simulink model "ITireAppMdl"  (R2017b)
settings: Solver=FixedStepDiscrete  StartTime=0.0  StopTime=10000  FixedStep=0.1  RelTol=1e-3
model workspace (MAT data in the model file):
  AilrflowValidFlag1 = [0.01235 0.03834 0.06233 0.08839 0.11261 0.13833 0.16348 0.18843 0.2134 0.23767 0.26241 0.28847 ... (108920 elements, 54460x2)]
  AilrflowValidFlag2 = [0.01258 0.03858 0.06256 0.08863 0.11285 0.13856 0.16371 0.18866 0.21363 0.2379 0.26264 0.2887 ... (108920 elements, 54460x2)]
  Airflow = [0.01258 0.03858 0.06256 0.08863 0.11285 0.13856 0.16371 0.18866 0.21363 0.2379 0.26264 0.2887 ... (108920 elements, 54460x2)]
  Frequency = [0.01235 0.03834 0.06233 0.08839 0.11261 0.13833 0.16348 0.18843 0.2134 0.23767 0.26241 0.28847 ... (108920 elements, 54460x2)]
  IntkAirHmdty = [0.07576 0.17591 0.27589 0.37591 0.47621 0.5753 0.67605 0.77531 0.87537 0.97532 1.07528 1.17533 ... (27230 elements, 13615x2)]
  IntkAirTemp = [0.07576 0.17591 0.27589 0.37591 0.47621 0.5753 0.67605 0.77531 0.87537 0.97532 1.07528 1.17533 ... (27230 elements, 13615x2)]
  IntkHmdtyTemp = [0.07576 0.17591 0.27589 0.37591 0.47621 0.5753 0.67605 0.77531 0.87537 0.97532 1.07528 1.17533 ... (27230 elements, 13615x2)]
  PriPresFilterValue = [0.01235 0.03834 0.06233 0.08839 0.11261 0.13833 0.16348 0.18843 0.2134 0.23767 0.26241 0.28847 ... (108920 elements, 54460x2)]
  PriPresRawValue = [0.01235 0.03834 0.06233 0.08839 0.11261 0.13833 0.16348 0.18843 0.2134 0.23767 0.26241 0.28847 ... (108920 elements, 54460x2)]
  SecPresFilterValue = [0.01258 0.03858 0.06256 0.08863 0.11285 0.13856 0.16371 0.18866 0.21363 0.2379 0.26264 0.2887 ... (108920 elements, 54460x2)]
  SecPresRawValue = [0.01258 0.03858 0.06256 0.08863 0.11285 0.13856 0.16371 0.18866 0.21363 0.2379 0.26264 0.2887 ... (108920 elements, 54460x2)]
  deltaPriPresFilterV = [0.01235 0.03834 0.06233 0.08839 0.11261 0.13833 0.16348 0.18843 0.2134 0.23767 0.26241 0.28847 ... (108920 elements, 54460x2)]
  deltaPriPresRawValu = [0.01235 0.03834 0.06233 0.08839 0.11261 0.13833 0.16348 0.18843 0.2134 0.23767 0.26241 0.28847 ... (108920 elements, 54460x2)]
  deltaSecPresFilterV = [0.01258 0.03858 0.06256 0.08863 0.11285 0.13856 0.16371 0.18866 0.21363 0.2379 0.26264 0.2887 ... (108920 elements, 54460x2)]
  deltaSecPresRawValu = [0.01258 0.03858 0.06256 0.08863 0.11285 0.13856 0.16371 0.18866 0.21363 0.2379 0.26264 0.2887 ... (108920 elements, 54460x2)]
values from neighbouring files (symbols this model uses):
  pTireHighPreDWLimit = 335.0    [ITiremyDictionary.sldd]
  pTireHighPreUpLimit = 350.0    [ITiremyDictionary.sldd]
  pTireLowPreDWLimit = 180.0    [ITiremyDictionary.sldd]
  pTireLowPreUpLimit = 195.0    [ITiremyDictionary.sldd]
(part 2 of 2)

== stateflow chart ITireAppMdl/High_Low_PrsERR ==
  (default) -> (junction 814)
  (junction 814) -> (junction 815) [order 1] : [TireLFPrs>TireLFPrsRef]
  (junction 814) -> (junction 809) [order 2]
  (junction 815) -> (junction 813) : {TireLFPrsRef=TireLFPrs;
      | TireLFPrsSlowCounts=0;}
  (junction 813) -> (junction 809)
  (junction 809) -> (junction 802)
  (junction 802) -> (junction 807) [order 1] : [TireLRPrs>TireLRPrsRef]
  (junction 802) -> (junction 801) [order 2]
  (junction 807) -> (junction 800) : {TireLRPrsRef=TireLRPrs;
      | TireLRPrsSlowCounts=0;}
  (junction 800) -> (junction 801)
  (junction 801) -> (junction 792)
  (junction 792) -> (junction 798) [order 1] : [TireRFPrs>TireRFPrsRef]
  (junction 792) -> (junction 793) [order 2]
  (junction 798) -> (junction 795) : {TireRFPrsRef=TireRFPrs;
      | TireRFPrsSlowCounts=0;}
  (junction 795) -> (junction 793)
  (junction 793) -> (junction 783)
  (junction 783) -> (junction 785) [order 1] : [TireRRPrs>TireRRPrsRef]
  (junction 783) -> (junction 781) [order 2]
  (junction 785) -> (junction 787) : {TireRRPrsRef=TireRRPrs;
      | TireRRPrsSlowCounts=0;}
  (junction 787) -> (junction 781)
  (junction 781) -> (junction 148)
  (junction 148) -> (junction 152) [order 1] : [TireRFPrsV==0]
  (junction 152) -> (junction 174) [order 1] : [TireRFPrs>pTireLowPreUpLimit]
  (junction 148) -> (junction 150) [order 2] : {RFTirePreStaus=3;}
  (junction 152) -> (junction 158) [order 2]
  (junction 174) -> (junction 176) : {RFTirePreStaus=0;}
  (junction 176) -> (junction 158)
  (junction 158) -> (junction 210)
  (junction 210) -> (junction 213) [order 1] : [TireRFPrs<pTireHighPreDWLimit]
  (junction 210) -> (junction 208) [order 2]
  (junction 213) -> (junction 209) : {RFTirePreStaus=0;}
  (junction 209) -> (junction 208)
  (junction 208) -> (junction 222)
  (junction 222) -> (junction 225) [order 1] : [TireRFPrs<pTireLowPreDWLimit]
  (junction 222) -> (junction 220) [order 2]
  (junction 225) -> (junction 221) : {RFTirePreStaus=2;}
  (junction 221) -> (junction 220)
  (junction 220) -> (junction 226)
  (junction 226) -> (junction 233) [order 1] : [TireRFPrs>pTireHighPreUpLimit]
  (junction 226) -> (junction 231) [order 2]
  (junction 233) -> (junction 232) : {RFTirePreStaus=1;}
  (junction 231) -> (junction 150)
  (junction 232) -> (junction 231)
  (junction 150) -> (junction 242)
  (junction 242) -> (junction 241) [order 1] : [TireLFPrsV==0]
  (junction 241) -> (junction 256) [order 1] : [TireLFPrs>pTireLowPreUpLimit]
  (junction 242) -> (junction 240) [order 2] : {LFTirePreStaus=3;}
  (junction 241) -> (junction 276) [order 2]
  (junction 256) -> (junction 237) : {LFTirePreStaus=0;}
  (junction 237) -> (junction 276)
  (junction 276) -> (junction 251)
  (junction 251) -> (junction 254) [order 1] : [TireLFPrs<pTireHighPreDWLimit]
  (junction 251) -> (junction 249) [order 2]
  (junction 254) -> (junction 250) : {LFTirePreStaus=0;}
  (junction 250) -> (junction 249)
  (junction 249) -> (junction 258)
  (junction 258) -> (junction 265) [order 1] : [TireLFPrs<pTireLowPreDWLimit]
  (junction 258) -> (junction 263) [order 2]
  (junction 265) -> (junction 264) : {LFTirePreStaus=2;}
  (junction 264) -> (junction 263)
  (junction 263) -> (junction 267)
  (junction 267) -> (junction 274) [order 1] : [TireLFPrs>pTireHighPreUpLimit]
  (junction 267) -> (junction 272) [order 2]
  (junction 274) -> (junction 273) : {LFTirePreStaus=1;}
  (junction 272) -> (junction 240)
  (junction 273) -> (junction 272)
  (junction 240) -> (junction 285)
  (junction 285) -> (junction 284) [order 1] : [TireLRPrsV==0]
  (junction 284) -> (junction 289) [order 1] : [TireLRPrs>pTireLowPreUpLimit]
  (junction 285) -> (junction 280) [order 2] : {LRTirePreStaus=3;}
  (junction 284) -> (junction 306) [order 2]
  (junction 289) -> (junction 279) : {LRTirePreStaus=0}
  (junction 279) -> (junction 306)
  (junction 306) -> (junction 291)
  (junction 291) -> (junction 293) [order 1] : [TireLRPrs<pTireHighPreDWLimit]
  (junction 291) -> (junction 298) [order 2]
  (junction 293) -> (junction 295) : {LRTirePreStaus=0}
  (junction 295) -> (junction 298)
  (junction 298) -> (junction 300)
  (junction 300) -> (junction 315) [order 1] : [TireLRPrs<pTireLowPreDWLimit]
  (junction 300) -> (junction 313) [order 2]
  (junction 315) -> (junction 316) : {LRTirePreStaus=2}
  (junction 316) -> (junction 313)
  (junction 313) -> (junction 318)
  (junction 318) -> (junction 309) [order 1] : [TireLRPrs>pTireHighPreUpLimit]
  (junction 318) -> (junction 312) [order 2]
  (junction 309) -> (junction 307) : {LRTirePreStaus=1}
  (junction 312) -> (junction 280)
  (junction 307) -> (junction 312)
  (junction 280) -> (junction 327)
  (junction 327) -> (junction 326) [order 1] : [TireRRPrsV==0]
  (junction 326) -> (junction 334) [order 1] : [TireRRPrs>pTireLowPreUpLimit]
  (junction 327) -> (junction 322) [order 2] : {LRTirePreStaus=3;}
  (junction 326) -> (junction 348) [order 2]
  (junction 334) -> (junction 321) : {RRTirePreStaus=0}
  (junction 321) -> (junction 348)
  (junction 348) -> (junction 331)
  (junction 331) -> (junction 340) [order 1] : [TireRRPrs<pTireHighPreDWLimit]
  (junction 331) -> (junction 338) [order 2]
  (junction 340) -> (junction 337) : {RRTirePreStaus=0}
  (junction 337) -> (junction 338)
  (junction 338) -> (junction 342)
  (junction 342) -> (junction 352) [order 1] : [TireRRPrs<pTireLowPreDWLimit]
  (junction 342) -> (junction 356) [order 2]
  (junction 352) -> (junction 347) : {RRTirePreStaus=2}
  (junction 347) -> (junction 356)
  (junction 356) -> (junction 360)
  (junction 360) -> (junction 349) [order 1] : [TireRRPrs>pTireHighPreUpLimit]
  (junction 360) -> (junction 355) [order 2]
  (junction 349) -> (junction 358) : {RRTirePreStaus=1}
  (junction 355) -> (junction 322)
  (junction 358) -> (junction 355)
  (junction 322) -> (junction 362)
  (junction 362) -> (junction 543)
  (junction 543) -> (junction 545) : {Time1SCount++;}
  (junction 545) -> (junction 547) [order 1] : [Time1SCount>=60]
  (junction 545) -> (junction 687) [order 2]
  (junction 547) -> (junction 549) : {Time1SCount=0;
      | i=59;}
  (junction 549) -> (junction 557)
  (junction 561) -> (junction 549) [order 1] : [i>=1]
  (junction 557) -> (junction 559) : {LFPress1MinArray[i]=LFPress1MinArray[i-1];
      | LFPressV1MinArray[i]=LFPressV1MinArray[i-1];
      | i--;}
  (junction 559) -> (junction 561)
  (junction 561) -> (junction 566) [order 2] : {LFPress1MinArray[0]=TireLFPrs;
      | LFPressV1MinArray[0]=TireLFPrsV;
      | i=1;
      | }
  (junction 566) -> (junction 706) [order 1] : [(TireLFPrsV==0)]
  (junction 706) -> (junction 571)
  (junction 571) -> (junction 693) [order 1] : [((LFPress1MinArray[i]-LFPress1MinArray[0])>20)&(TireLFPrs>pTireLowPreDWLimit)]
  (junction 566) -> (junction 573) [order 2] : {LFTireLeakStaus=3;}
  (junction 715) -> (junction 706)
  (junction 571) -> (junction 708) [order 2] : {i++}
  (junction 693) -> (junction 701) : {LFTireLeakStaus=1;
      | TireLFPrsRef=TireLFPrs;
      | TireLFPrsSlowCounts=0;}
  (junction 708) -> (junction 715) [order 1] : [i<=59]
  (junction 708) -> (junction 703) [order 2] : {LFTireLeakStaus=0;}
  (junction 703) -> (junction 573)
  (junction 701) -> (junction 703)
  (junction 573) -> (junction 608) : {i=59;}
  (junction 608) -> (junction 611)
  (junction 609) -> (junction 608) [order 1] : [i>=1]
  (junction 611) -> (junction 613) : {LRPress1MinArray[i]=LRPress1MinArray[i-1];
      | LRPressV1MinArray[i]=LRPressV1MinArray[i-1];
      | i--;}
  (junction 613) -> (junction 609)
  (junction 609) -> (junction 605) [order 2] : {LRPress1MinArray[0]=TireLRPrs;
      | LRPressV1MinArray[0]=TireLRPrsV;
      | i=1;}
  (junction 605) -> (junction 724) [order 1] : [(TireLRPrsV==0)]
  (junction 724) -> (junction 722)
  (junction 722) -> (junction 735) [order 1] : [((LRPress1MinArray[i]-LRPress1MinArray[0])>20)&(TireLRPrs>pTireLowPreDWLimit)]
  (junction 605) -> (junction 600) [order 2] : {LRTireLeakStaus=3;}
  (junction 732) -> (junction 724)
  (junction 722) -> (junction 727) [order 2] : {i++}
  (junction 735) -> (junction 734) : {LRTireLeakStaus=1;
      | TireLRPrsRef=TireLRPrs;
      | TireLRPrsSlowCounts=0;}
  (junction 727) -> (junction 732) [order 1] : [i<=59]
  (junction 727) -> (junction 725) [order 2] : {LRTireLeakStaus=0;}
  (junction 734) -> (junction 725)
  (junction 725) -> (junction 600)
  (junction 600) -> (junction 634) : {i=59;}
  (junction 634) -> (junction 637)
  (junction 635) -> (junction 634) [order 1] : [i>=1]
  (junction 637) -> (junction 639) : {RFPress1MinArray[i]=RFPress1MinArray[i-1];
      | RFPressV1MinArray[i]=RFPressV1MinArray[i-1];
      | i--;}
  (junction 639) -> (junction 635)
  (junction 635) -> (junction 631) [order 2] : {RFPress1MinArray[0]=TireRFPrs;
      | RFPressV1MinArray[0]=TireRFPrsV;
      | i=1;}
  (junction 631) -> (junction 744) [order 1] : [(TireRFPrsV==0)]
  (junction 744) -> (junction 739)
  (junction 739) -> (junction 749) [order 1] : [((RFPress1MinArray[i]-RFPress1MinArray[0])>20)&(TireRFPrs>pTireLowPreDWLimit)]
  (junction 631) -> (junction 626) [order 2] : {RFTireLeakStaus=3;}
  (junction 752) -> (junction 744)
  (junction 739) -> (junction 746) [order 2] : {i++}
  (junction 749) -> (junction 751) : {RFTireLeakStaus=1;
      | TireRFPrsRef=TireRFPrs;
      | TireRFPrsSlowCounts=0;}
  (junction 746) -> (junction 752) [order 1] : [i<=59]
  (junction 746) -> (junction 742) [order 2] : {RFTireLeakStaus=0;}
  (junction 751) -> (junction 742)
  (junction 742) -> (junction 626)
  (junction 626) -> (junction 647) : {i=59;}
  (junction 647) -> (junction 663)
  (junction 661) -> (junction 647) [order 1] : [i>=1]
  (junction 663) -> (junction 665) : {RRPress1MinArray[i]=RRPress1MinArray[i-1];
      | RRPressV1MinArray[i]=RRPressV1MinArray[i-1];
      | i--;}
  (junction 665) -> (junction 661)
  (junction 661) -> (junction 657) [order 2] : {RRPress1MinArray[0]=TireRRPrs;
      | RRPressV1MinArray[0]=TireRRPrsV;}
  (junction 657) -> (junction 767) [order 1] : [(TireRRPrsV==0)]
  (junction 767) -> (junction 757)
  (junction 757) -> (junction 768) [order 1] : [((RRPress1MinArray[i]-RRPress1MinArray[0])>20)&(TireRRPrs>pTireLowPreDWLimit)]
  (junction 657) -> (junction 652) [order 2] : {RRTireLeakStaus=3;}
  (junction 760) -> (junction 767)
  (junction 757) -> (junction 765) [order 2] : {i++}
  (junction 768) -> (junction 759) : {RRTireLeakStaus=1;
      | TireRRPrsRef=TireRRPrs;
      | TireRRPrsSlowCounts=0;}
  (junction 765) -> (junction 760) [order 1] : [i<=59]
  (junction 765) -> (junction 769) [order 2] : {RRTireLeakStaus=0;}
  (junction 759) -> (junction 769)
  (junction 769) -> (junction 652)
  (junction 652) -> (junction 673)
  (junction 673) -> (junction 818) [order 1] : [(TireLFPrs<=TireLFPrsRef)&&(LFTireLeakStaus==0)]
  (junction 673) -> (junction 836) [order 2]
  (junction 818) -> (junction 820) : {TireLFPrsSlowCounts++;}
  (junction 820) -> (junction 824) [order 1] : [(TireLFPrsSlowCounts<36000)&&((TireLFPrsRef-TireLFPrs)>25)&&(TireLFPrs>pTireLowPreDWLimit)]
  (junction 820) -> (junction 826) [order 2] : {LFTireLeakStaus=0;}
  (junction 824) -> (junction 828) : {LFTireLeakStaus=2;
      | TireSlowLifeLF=((TireLFPrsRef-pTireLowPreDWLimit)/(TireLFPrsRef-TireLFPrs))*(TireLFPrsSlowCounts/600);}
  (junction 826) -> (junction 831) [order 1] : [(TireLFPrsSlowCounts>=36000)]
  (junction 826) -> (junction 839) [order 2]
  (junction 831) -> (junction 832) : {TireLFPrsSlowCounts=0;
      | TireLFPrsRef=TireLFPrs}
  (junction 839) -> (junction 836)
  (junction 832) -> (junction 839)
  (junction 828) -> (junction 832)
  (junction 836) -> (junction 843)
  (junction 843) -> (junction 853) [order 1] : [(TireLRPrs<=TireLRPrsRef)&(LRTireLeakStaus==0)]
  (junction 843) -> (junction 852) [order 2]
  (junction 853) -> (junction 848) : {TireLRPrsSlowCounts++;}
  (junction 848) -> (junction 865) [order 1] : [(TireLRPrsSlowCounts<36000)&((TireLRPrsRef-TireLRPrs)>25)&(TireLRPrs>pTireLowPreDWLimit)]
  (junction 848) -> (junction 850) [order 2] : {LRTireLeakStaus=0}
  (junction 865) -> (junction 847) : {LRTireLeakStaus=2;
      | TireSlowLifeLR=((TireLRPrsRef-pTireLowPreDWLimit)/(TireLRPrsRef-TireLRPrs))*(TireLRPrsSlowCounts/600);}
  (junction 850) -> (junction 857) [order 1] : [(TireLRPrsSlowCounts>=36000)]
  (junction 850) -> (junction 846) [order 2]
  (junction 857) -> (junction 862) : {TireLRPrsSlowCounts=0;
      | TireLRPrsRef=TireLFPrs}
  (junction 846) -> (junction 852)
  (junction 862) -> (junction 846)
  (junction 847) -> (junction 862)
  (junction 852) -> (junction 868)
  (junction 868) -> (junction 875) [order 1] : [(TireRFPrs<=TireRFPrsRef)&(RFTireLeakStaus==0)]
  (junction 868) -> (junction 882) [order 2]
  (junction 875) -> (junction 866) : {TireRFPrsSlowCounts++}
  (junction 866) -> (junction 887) [order 1] : [(TireRFPrsSlowCounts<36000)&((TireRFPrsRef-TireRFPrs)>25)&(TireRFPrs>pTireLowPreDWLimit)]
  (junction 866) -> (junction 873) [order 2] : {RFTireLeakStaus=0}
  (junction 887) -> (junction 870) : {RFTireLeakStaus=2;
      | TireSlowLifeRF=((TireRFPrsRef-pTireLowPreDWLimit)/(TireRFPrsRef-TireRFPrs))*(TireRFPrsSlowCounts/600);}
  (junction 873) -> (junction 878) [order 1] : [(TireRFPrsSlowCounts>=36000)]
  (junction 873) -> (junction 869) [order 2]
  (junction 878) -> (junction 872) : {TireRFPrsSlowCounts=0;
      | TireRFPrsRef=TireLFPrs}
  (junction 869) -> (junction 882)
  (junction 872) -> (junction 869)
  (junction 870) -> (junction 872)
  (junction 882) -> (junction 894)
  (junction 894) -> (junction 893) [order 1] : [(TireRRPrs<=TireRRPrsRef)&(RRTireLeakStaus==0)]
  (junction 894) -> (junction 904) [order 2]
  (junction 893) -> (junction 889) : {TireRRPrsSlowCounts++}
  (junction 889) -> (junction 910) [order 1] : [(TireRRPrsSlowCounts<36000)&((TireRRPrsRef-TireRRPrs)>25)&(TireRRPrs>pTireLowPreDWLimit)]
  (junction 889) -> (junction 895) [order 2] : {RRTireLeakStaus=0 }
  (junction 910) -> (junction 897) : {RRTireLeakStaus=2;
      | TireSlowLifeRR=((TireRRPrsRef-pTireLowPreDWLimit)/(TireRRPrsRef-TireRRPrs))*(TireRRPrsSlowCounts/600);}
  (junction 895) -> (junction 901) [order 1] : [(TireRRPrsSlowCounts>=36000)]
  (junction 895) -> (junction 898) [order 2]
  (junction 901) -> (junction 896) : {TireRRPrsSlowCounts=0;
      | TireRRPrsRef=TireLFPrs;}
  (junction 904) -> (junction 687)
  (junction 898) -> (junction 904)
  (junction 896) -> (junction 898)
  (junction 897) -> (junction 896)
  data: TireRFPrsV input uint8 [0..1]; TireLFPrsV input uint8 [0..1]; TireRRPrsV input uint8 [0..1]; TireLRPrsV input uint8 [0..1]; TireLFPrs input uint16 [0..1]; TireLRPrs input uint16 [0..1]; TireRFPrs input uint16 [0..1]; TireRRPrs input uint16 [0..1]; pTireHighPreUpLimit parameter double; pTireHighPreDWLimit parameter double; pTireLowPreUpLimit parameter double; pTireLowPreDWLimit parameter double; RFTirePreStaus output uint8; LFTirePreStaus output uint8; LRTirePreStaus output uint8; RRTirePreStaus output uint8; LFTireLeakStaus output uint8 =0; LRTireLeakStaus output uint8 =0; RFTireLeakStaus output uint8 =0; RRTireLeakStaus output uint8 =0; LFPress1MinArray local uint16 size=[1 60] =0; Time1SCount local uint8 =10; i local uint8 =0; LFPressV1MinArray local uint8 size=[1 60] =0; LRPressV1MinArray local uint8 size=[1 60] =0; RFPressV1MinArray local uint8 size=[1 60] =0; RRPressV1MinArray local uint8 size=[1 60] =0; RFPress1MinArray local uint16 size=[1 60] =0; LRPress1MinArray local uint16 size=[1 60] =0; RRPress1MinArray local uint16 size=[1 60] =0; TireLFPrsRef local uint16 [0..1] =0; TireLRPrsRef local uint16 [0..1] =0; TireRFPrsRef local uint16 [0..1] =0; TireRRPrsRef local uint16 [0..1] =0; TireLFPrsSlowCounts local uint16 [0..1] =0; TireLRPrsSlowCounts local uint16 [0..1] =0; TireRRPrsSlowCounts local uint16 [0..1] =0; TireSlowLifeLF output uint8; TireRFPrsSlowCounts local uint16 [0..1] =0; TireSlowLifeLR output uint8; TireSlowLifeRF output uint8; TireSlowLifeRR output uint8

== stateflow chart ITireAppMdl/TireTempStatus ==
  (default) -> (junction 13)
  (junction 13) -> (junction 19) [order 1] : [TireLFTmpV==0]
  (junction 19) -> (junction 21) [order 1] : [TireLFTmp>70]
  (junction 13) -> (junction 17) [order 2] : {LFTireTempStaus=3;}
  (junction 19) -> (junction 24) [order 2] : {LFTireTempStaus=0;}
  (junction 21) -> (junction 25) : {LFTireTempStaus=1;}
  (junction 24) -> (junction 17)
  (junction 25) -> (junction 24)
  (junction 17) -> (junction 30)
  (junction 30) -> (junction 33) [order 1] : [TireLRTmpV==0]
  (junction 33) -> (junction 42) [order 1] : [TireLRTmp>70]
  (junction 30) -> (junction 36) [order 2] : {LRTireTempStaus=3;}
  (junction 33) -> (junction 37) [order 2] : {LRTireTempStaus=0;}
  (junction 42) -> (junction 43) : {LRTireTempStaus=1;}
  (junction 37) -> (junction 36)
  (junction 43) -> (junction 37)
  (junction 36) -> (junction 48)
  (junction 48) -> (junction 55) [order 1] : [TireRFTmpV==0]
  (junction 55) -> (junction 51) [order 1] : [TireRFTmp>70]
  (junction 48) -> (junction 58) [order 2] : {RFTireTempStaus=3;}
  (junction 55) -> (junction 45) [order 2] : {RFTireTempStaus=0;}
  (junction 51) -> (junction 46) : {RFTireTempStaus=1;}
  (junction 45) -> (junction 58)
  (junction 46) -> (junction 45)
  (junction 58) -> (junction 66)
  (junction 66) -> (junction 70) [order 1] : [TireRRTmpV==0]
  (junction 70) -> (junction 67) [order 1] : [TireRRTmp>70]
  (junction 66) -> (junction 72) [order 2] : {RRTireTempStaus=3;}
  (junction 70) -> (junction 61) [order 2] : {RRTireTempStaus=0;}
  (junction 67) -> (junction 60) : {RRTireTempStaus=1;}
  (junction 61) -> (junction 72)
  (junction 60) -> (junction 61)
  (junction 72) -> (junction 75)
  data: TireLFTmpV input uint8; TireLFTmp input int16; TireLRTmpV input uint8; TireLRTmp input int16; TireRFTmpV input uint8; TireRFTmp input int16; TireRRTmpV input uint8; TireRRTmp input int16; LFTireTempStaus output uint8; LRTireTempStaus output uint8; RFTireTempStaus output uint8; RRTireTempStaus output uint8; data local double

== stateflow chart ITireAppMdl/SensorLostERR ==
  (default) -> (junction 16)
  (junction 16) -> (junction 22) [order 2] : {LFTirPreSenLostErrV=0;
      | LRTirPreSenLostErrV=0;RFTirPreSenLostErrV=0;
      | RRTirPreSenLostErrV=0;}
  (junction 22) -> (junction 26) [order 2] : {TireRFPrsLostCount=0;}
  (junction 16) -> (junction 18) [order 1] : [(VehSpdAvgNDrvn<37)||(VehSpdAvgNDrvnV==1)]{LFTirPreSenLostErrV=1;
      | LRTirPreSenLostErrV=1;RFTirPreSenLostErrV=1;
      | RRTirPreSenLostErrV=1;}
  (junction 22) -> (junction 24) [order 1] : [TireRFPrsV==1]{TireRFPrsLostCount = TireRFPrsLostCount + 1;}
  (junction 26) -> (junction 28)
  (junction 28) -> (junction 24)
  (junction 24) -> (junction 33)
  (junction 33) -> (junction 118) [order 2] : {TireLFPrsLostCount=0;}
  (junction 33) -> (junction 47) [order 1] : [TireLFPrsV==1]{TireLFPrsLostCount = TireLFPrsLostCount + 1;}
  (junction 118) -> (junction 120)
  (junction 120) -> (junction 47)
  (junction 47) -> (junction 55)
  (junction 55) -> (junction 129) [order 2] : {TireLRPrsLostCount=0;}
  (junction 55) -> (junction 63) [order 1] : [TireLRPrsV==1]{TireLRPrsLostCount = TireLRPrsLostCount + 1;}
  (junction 129) -> (junction 130)
  (junction 130) -> (junction 63)
  (junction 63) -> (junction 70)
  (junction 70) -> (junction 134) [order 2] : {TireRRPrsLostCount=0;}
  (junction 70) -> (junction 69) [order 1] : [TireRRPrsV==1]{TireRRPrsLostCount = TireRRPrsLostCount + 1;}
  (junction 134) -> (junction 135)
  (junction 135) -> (junction 69)
  (junction 69) -> (junction 73)
  (junction 73) -> (junction 77) [order 2] : {RFTirPreSenLostErr=0;}
  (junction 73) -> (junction 75) [order 1] : [TireRFPrsLostCount>pTirePrsLostCountTh]{RFTirPreSenLostErr=1;
      | TireRFPrsLostCount=pTirePrsLostCountTh}
  (junction 77) -> (junction 79)
  (junction 79) -> (junction 75)
  (junction 75) -> (junction 84)
  (junction 84) -> (junction 82) [order 2] : {LFTirPreSenLostErr=0;}
  (junction 84) -> (junction 90) [order 1] : [TireLFPrsLostCount>pTirePrsLostCountTh]{LFTirPreSenLostErr=1;
      | TireLFPrsLostCount=pTirePrsLostCountTh}
  (junction 82) -> (junction 88)
  (junction 88) -> (junction 90)
  (junction 90) -> (junction 98)
  (junction 98) -> (junction 99) [order 2] : {LRTirPreSenLostErr=0;}
  (junction 98) -> (junction 92) [order 1] : [TireLRPrsLostCount>pTirePrsLostCountTh]{LRTirPreSenLostErr=1;
      | TireLRPrsLostCount=pTirePrsLostCountTh}
  (junction 99) -> (junction 93)
  (junction 93) -> (junction 92)
  (junction 92) -> (junction 107)
  (junction 107) -> (junction 102) [order 2] : {RRTirPreSenLostErr=0;}
  (junction 107) -> (junction 103) [order 1] : [TireRRPrsLostCount>pTirePrsLostCountTh]{RRTirPreSenLostErr=1;
      | TireRRPrsLostCount=pTirePrsLostCountTh}
  (junction 102) -> (junction 106)
  (junction 106) -> (junction 103)
  (junction 103) -> (junction 109)
  (junction 109) -> (junction 18)
  data: TireRFPrsV input uint8 [0..1]; TireLFPrsV input uint8 [0..1]; TireRRPrsV input uint8 [0..1]; TireLRPrsV input uint8 [0..1]; TireLFPrs input uint16 [0..1]; TireLRPrs input uint16 [0..1]; TireRFPrs input uint16 [0..1]; TireRRPrs input uint16 [0..1]; LFTirPreSenLostErr output uint8; LFTirPreSenLostErrV output uint8 [0..1]; VehSpdAvgNDrvn input double; VehSpdAvgNDrvnV input uint8; pTirePrsLostCountTh parameter double; LRTirPreSenLostErr output uint8; RFTirPreSenLostErr output uint8; RRTirPreSenLostErr output uint8; LRTirPreSenLostErrV output uint8 [0..1]; RFTirPreSenLostErrV output uint8 [0..1]; RRTirPreSenLostErrV output uint8 [0..1]; TireRFPrsLostCount local uint16 size=1 =0; TireLFPrsLostCount local uint16 size=1 =0; TireLRPrsLostCount local uint16 size=1 =0; TireRRPrsLostCount local uint16 size=1 =0
